simulink model "EMC_no_hand"  (R2015a)
settings: Solver=ode4  SolverMode=MultiTasking  StartTime=0.0  StopTime=inf  FixedStep=BKIN_STEP_TIME  RelTol=1e-3
StartFcn:
  |  warndlg('Dexterit-E models cannot run under simulation. Please compile your model and run it from within Dexterit-E.');set_param(bdroot,'SimulationCommand','stop')
model workspace (MAT data in the model file):
  BKIN_KINEMATIC_FRAME_SIZE = 400
  BKIN_STEP_TIME = 0.00025
  COLOR = 4
  COL_X = 1
  COL_Y = 2
  E_NO_EVENT = 0
  LOAD_X = 1
  LOAD_Y = 2
  MOVEMENT_DELAY = 3
  PATH_LENGTH = 1
  PATH_PERIOD = 2
  POST_TRIAL_DELAY = 4
  RADIUS = 3
  TRAJECTORY = 1
  TRAJECTORY_TYPE = 2
  TRIAL_END = 3
  TRIAL_MOVEMENT = 2
  TRIAL_RESET = 4
  TRIAL_START = 1
  X_POSITION = 1
  Y_POSITION = 2
  col_x = 1
  col_y = 2
  ANGULAR_THRESHOLD = 5
  GAZE_EXIT = 6
  START_REACHED = 7
  FIXATION_DURATION = 6
  TRACKING_TARGET_ROW = 7
  FEEDBACK_COLOR = 5
  CROSS_LOGICAL_RADIUS = 8
  DETECT_FIXATION = 8
  GAZE_IN_TARGET = 5
  START_STABILIZATION = 9
  HAND_IN_TARGET = 9
  BACKGROUND_LOAD = 10
  DIST_BETWEEN_TRAJ = 11
  STRAIGHT_PAUSE_TIME = 12
libraries: simulink x14, xpcrtudplib x12, xpcutilitieslib x10, xpcobsoletelib x8, slrtlib x2, ethercat x2, General x2, Video x2
(part 1 of 6)
settings Model: ModifiedComment=chris -- Wed Feb 16 09:18:30 2005 -- Version 1.1384  ModifiedHistory=Feb 16/05 - Add error repeat, add offset ramp  CovHtmlReporting=off  ExtModeArmWhenConnect=off  ExtModeLogAll=off  Creator=Chris Grebeldinger  LastModifiedBy=Brain and Action Lab
settings SolverCC: EnableConcurrentExecution=on  AutoInsertRateTranBlk=on
settings DataIOCC: LimitDataPoints=off  SignalLoggingSaveFormat=ModelDataLogs  SaveOutput=off  SaveTime=off  SignalLoggingName=sigsOut
settings OptimizationCC: BlockReduction=off  BooleanDataType=off  OptimizeBlockIOStorage=off  BufferReuse=off  GlobalBufferReuse=off  ExpressionFolding=off  ExpressionDepthLimit=2147483647  LocalBlockOutputs=off  InitFltsAndDblsToZero=on
settings DebuggingCC: SaveWithParameterizedLinksMsg=none  UnderspecifiedInitializationDetection=Classic  MergeDetectMultiDrivingBlocksExec=none  SignalResolutionControl=TryResolveAllWithWarning  MultiTaskDSMMsg=warning  FcnCallInpInsideContextMsg=EnableAllAsWarning  StateNameClashWarn=warning  StrictBusMsg=ErrorOnBusTreatedAsVector
settings HardwareCC: ProdIntDivRoundTo=Zero  ProdEndianess=LittleEndian  ProdLongLongMode=on  ProdHWDeviceType=Generic->32-bit x86 compatible  TargetHWDeviceType=32-bit Generic
settings SFSimCC: SimCustomSourceCode=#include <stdlib.h>  SimCustomHeaderCode="#include \"stdlib.h\""  SFSimEcho=off  SimParseCustomCode=off
settings RTWCC: SystemTargetFile=slrt.tlc  TemplateMakefile=slrt_default_tmf  Description=Simulink Real-Time  CustomSourceCode="#include \"stdlib.h\""  CodeExecutionProfiling=on
settings CodeAppCC: MaxIdLength=63
settings SimulinkRealTimeCC: TargetFcnLib=ansi_tfl_tmw.mat  GeneratePreprocessorConditionals=Disable all

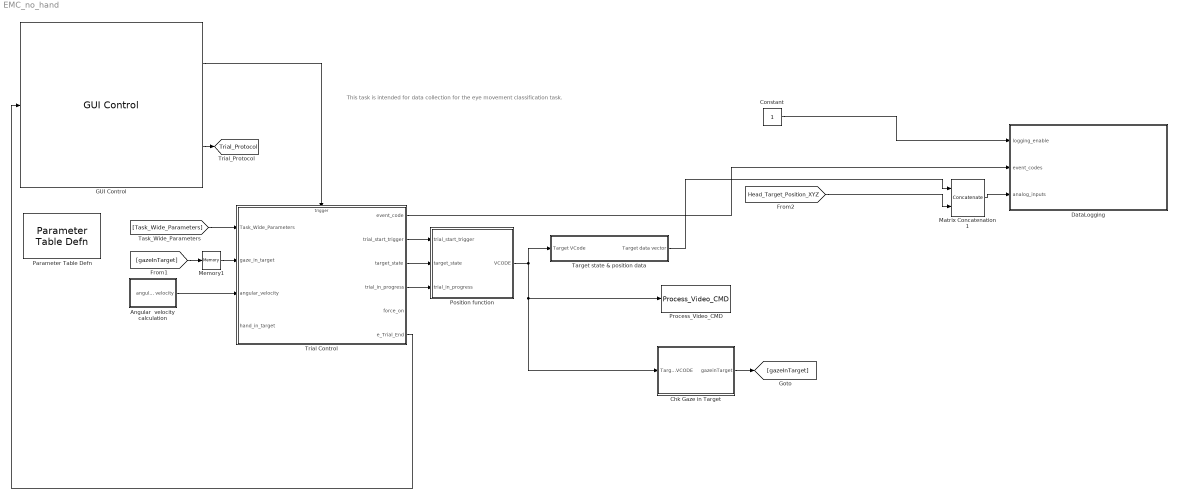
== system EMC_no_hand ==
  note: This task is intended for data collection for the eye movement classification task.
  Angular  velocity calculation : Subsystem
  Chk Gaze in Target : Subsystem
  Constant : Constant
  DataLogging : Subsystem  AncestorBlock=General/DataLogging  mask(DataLogging){log_event_codes=on, log_analog_inputs=on, show_time_remaining=off, ecat_include=on}
      mask prompts: log_event_codes "Log event codes"; log_analog_inputs "Log analog inputs"; show_time_remaining "Show time remaining"; ecat_include "Include EtherCAT control"
      mask help:
      | <b>Do not rename this block, it must be called 'DataLogging'.</b>
      | <p>
      | This block collects the following data and sends it to Dexterit-E:
      | <ul>
      | <li>Robot kinematics</li>
      | <li>Data from KINARM Lab peripherals (optional)</li>
      | <li>Event codes (optional)</li>
      | <li>Programmer supplied data and analog inputs (optional)</li>
      | <li>Remaining task time in seconds (optional)</li>
      | <li>Including code for EtherCAT control system (optional)</li>
      | </lu>
      | <p>
      | This block must be present in all task programs.
      mask init:
      | %this stops us from running a simulation
      | set_param(bdroot,'StartFcn',' warndlg(''Dexterit-E models cannot run under simulation. Please compile your model and run it from within Dexterit-E.'');set_param(bdroot,''SimulationCommand'',''stop'')')
      | 
      | block_path = gcb;  % store block path, as gcb may change with block operations
      |  
      | idxs = findstr(block_path, '/DataLogging');
      | [idxCount, n] = size(idxs);
      | [m, strlen] = size(block_path);
      | bColorSet = 0;
      | 
      | dexcheck();
      | if idxCount == 0 || idxs(1) ~= strlen - 11
      |     fprintf('=========ERROR====================\n');
      |     fprintf('%s should be called DataLogging, attempting to rename.\n', block_path);
      |     try
      |         set_param(block_path, 'Name', 'DataLogging');
      |         block_path = gcb;  % store block path, as gcb may change with block operations
      |         fprintf('Rename successful\n');
      |     catch err
      |         fprintf('Rename failed. You may have 2 DataLogging blocks or another improperly named block.\n');
      |        	set_param(block_path, 'BackgroundColor', '[0.9, 0, 0]');
      |         bColorSet = 1;
      |     end
      |     fprintf('=============================\n');
      | end
      | 
      | log_event_codes = strcmp(get_param(block_path, 'log_event_codes'), 'on');
      | log_analog_inputs = strcmp(get_param(block_path, 'log_analog_inputs'), 'on');
      | show_time_remaining = strcmp(get_param(block_path, 'show_time_remaining'), 'on');
      | 
      | 
      | % Handle the event codes setting: swap the 'Event Codes' inport with a constant block or 
      | % vice versa, if necessary, so that it matches the setting.
      | block_type = get_param([block_path '/event_codes'], 'BlockType');
      |  
      | if log_event_codes && ~strcmp(block_type, 'Inport') || ...  % if a change is required...
      |    ~log_event_codes && strcmp(block_type, 'Inport')
      |     
      |     % ...delete the existing block, ...
      |     pos = get_param([block_path '/event_codes'], 'Position');
      |     delete_line(block_path, 'event_codes/1', 'Create Event Codes Subsystem/1');
      |     delete_block([block_path '/event_codes']);
      |     
      |     % ...add an Inport or a 0-value Constant in place of the previous block (according to
      |     % the new setting), update the signal width flag, and then...
      |     if log_event_codes && ~strcmp(block_type, 'Inport')
      |         add_block('built-in/Inport', [block_path '/event_codes'], 'Name', 'event_codes');
      |         set_param([block_path '/Create Event Codes Subsystem/Not Logging Event Codes'], 'Value', '0');
      |     else
      |         add_block('built-in/Constant', [block_path '/event_codes'], 'Name', 'event_codes');
      |         set_param([block_path '/event_codes'], 'Value', '0');
      |         set_param([block_path '/Create Event Codes Subsystem/Not Logging Event Codes'], 'Value', '1');
      |     end
      |     
      |     % ...connect the new block.
      |     set_param([block_path '/event_codes'], 'Position', pos);
      |     add_line(block_path, 'event_codes/1', 'Create Event Codes Subsystem/1');
      | end
      | 
      | % Swap the 'analog_data' inport with a constant block or vice versa according to the corresponding setting.
      | block_type = get_param([block_path '/analog_inputs'], 'BlockType');
      | 
      | if log_analog_inputs && ~strcmp(block_type, 'Inport') || ...  % if a change is required...
      |    ~log_analog_inputs && strcmp(block_type, 'Inport')
      |     
      |     % ...delete the existing block, ...
      |     pos = get_param([block_path '/analog_inputs'], 'Position');
      |     delete_line(block_path, 'analog_inputs/1', 'Create Analog Inputs Subsystem/1');
      |     delete_block([block_path '/analog_inputs']);
      |     
      |     % ...add an Inport or a 0-value Constant in place of the previous block (according to
      |     % the new setting), update the signal width flag, and then...
      |     if log_analog_inputs && ~strcmp(block_type, 'Inport')
      |         add_block('built-in/Inport', [block_path '/analog_inputs'], 'Name', 'analog_inputs');
      |         set_param([block_path '/Create Analog Inputs Subsystem/Not Logging Analog Inputs'], 'Value', '0');
      |     else
      |         add_block('built-in/Constant', [block_path '/analog_inputs'], 'Name', 'analog_inputs');
      |         set_param([block_path '/analog_inputs'], 'Value', '0');
      |         set_param([block_path '/Create Analog Inputs Subsystem/Not Logging Analog Inputs'], 'Value', '1');
      |     end
      |     
      |     % ...connect the new block.
      |     set_param([block_path '/analog_inputs'], 'Position', pos);
      |     add_line(block_path, 'analog_inputs/1', 'Create Analog Inputs Subsystem/1');
      | end
      | 
      | %%%%%%%%%%%%%%%%%%%%%%%%%%%%%%%%%%%%%%%%%%%%%
      | block_type = get_param([block_path '/seconds_remaining'], 'BlockType');
      |  
      | if show_time_remaining && ~strcmp(block_type, 'Inport') || ...  % if a change is required...
      |    ~show_time_remaining && strcmp(block_type, 'Inport')
      |     
      |     % ...delete the existing block, ...
      |     pos = get_param([block_path '/seconds_remaining'], 'Position');
      |     delete_line(block_path, 'seconds_remaining/1', 'Create Custom Data Subsystem/1');
      |     delete_block([block_path '/seconds_remaining']);
      |     
      |     % ...add an Inport or a 0-value Constant in place of the previous block (according to
      |     % the new setting), update the signal width flag, and then...
      |     if show_time_remaining && ~strcmp(block_type, 'Inport')
      |         add_block('built-in/Inport', [block_path '/seconds_remaining'], 'Name', 'seconds_remaining');
      |     else
      |         add_block('built-in/Constant', [block_path '/seconds_remaining'], 'Name', 'seconds_remaining');
      |         set_param([block_path '/seconds_remaining'], 'Value', '-1');
      |     end
      |     
      |     % ...connect the new block.
      |     set_param([block_path '/seconds_remaining'], 'Position', pos);
      |     add_line(block_path, 'seconds_remaining/1', 'Create Custom Data Subsystem/1');
      | end
      | %%%%%%%%%%%%%%%%%%%%%%%%%%%%%%%%%%%%%%%%%%%%%%%%%%%%%%%%%
      | 
      | % Create the text label for the block, and use it to create the first in a 
      | % list of drawing commands that will be used to draw the mask icon.
      | label = 'Logging:\n ';
      |  
      | if log_event_codes
      |    label = [label 'Event codes\n'];
      | end
      |  
      | label = [label 'KINARM data\n'];
      |     
      | if log_analog_inputs
      |     label = [label 'Analog inputs\n'];
      | end
      | 
      | if show_time_remaining
      |     label = [label 'Seconds remaining\n'];
      | end
      | 
      | draw_commands = 'disp(label); ';
      | 
      | % Ensure the inports appear in a fixed order, and for each inport found add
      | % to the list of drawing commands a command to label it.
      | inports = find_system(block_path, 'LookUnderMasks', 'all', 'FollowLinks', 'on', 'SearchDepth', 1, 'BlockType', 'Inport');
      | 
      | for i = 1:length(inports)
      |     inport_name = char(get_param(inports(i), 'Name'));
      |     
      |     if strcmp(inport_name, 'logging_enable')
      |         port = '1';
      |     elseif strcmp(inport_name, 'event_codes')
      |         port = '2';
      |     elseif strcmp(inport_name, 'analog_inputs')
      |         if log_event_codes
      |             port = '3';
      |         else
      |             port = '2';
      |         end
      |     elseif strcmp(inport_name, 'seconds_remaining')
      |         if log_event_codes && log_analog_inputs
      |             port = '4';
      |         elseif log_event_codes || log_analog_inputs
      |             port = '3';
      |         else
      |             port = '2';                
      |         end
      |     end
      |     
      |     set_param([block_path '/' inport_name], 'Port', port);
      |     draw_commands = [draw_commands 'port_label(''input'', ' port ', ''' inport_name '''); '];
      | end
      | 
      | % Apply the drawing commands.
      | set_param(block_path, 'MaskDisplay', draw_commands);
      | 
      | %%% Handle background colours if link status changes.  
      | checkBackgroundColour(block_path, 'General');
      | 
      | % For gaze tracking, the packet length is variable, so we need to check off that option the Receive UDP block.
      | %set_param([block_path '/Receive_Gaze/Receive'], 'vblLen', 'on')
      | 
      | updateUDP([block_path '/Network Transfer Subsystem/UDP Receiver']);
      | initPollKINARM(ecat_include);
      settings: PostSaveFcn=|
      | name_size = strfind(gcb, '/') - 1;
      | if name_size > 50
      |   warndlg('The given file name is longer than 50 characters. The task name will be truncated in Dexterit-E.')
      | end
      mask Help:
      | Sends task progress, kinematics, analog data and event codes to Dexterit-E.
      | 
      | <H2>Library </H2>
      | General
      | 
      | <H2>Description </H2>
      | <b>Do not rename this block, it must be called 'DataLogging'.</b>
      | <p>
      | The DataLogging block collects data and event codes and sends it to Dexterit-E for saving.  It also passes on Task Program information that is invisible to the user, and so must be present even if no data is going to be saved.
      | <P>
      | <B><I>This block must be present in all Task Programs, even if no data is going to be saved.</I></B>
      | 
      | 
      | <H2>Parameters and Dialog Box</H2>
      | <ul><li><B>Log event codes: </B> checking this parameter causes the Dexterit-E to log event codes specified by the event_codes input.
      | Event codes are only saved at 1 kHz. If you need to save event codes at a higher rate then you will need to send an array of values to the event_codes input.
      | </li>
      | <li><B>Log analog inputs: </B> checking this parameter causes Dexterit-E to log analog data specified by the analog_inputs input.
      | Analog data in this context can be any numbers you would like to save. The data can truly be analog data from a card like the NI-6229,
      | but it can also be calculations created during your model's execution. For example, if you move targets around the screen then it
      | can be useful to send the target X, Y positions out as 2 separate "analog channels".
      | </li>
      | <li><B>Show time remaining: </B> checking this parameter causes Dexterit-E to display the number of seconds remaining in the task as specified by the seconds_remaining input
      | </li>
      | <li><b>Include EtherCAT control: </b>KINARM labs have one of two different control systems: PMAC or EtherCAT. If your KINARM uses the PMAC control system AND you are not planning to run your task on KINARMs that use the EtherCAT control system then you can uncheck this box. You can find out which control system your KINARM uses by looking in Dexterit-E at the "KINARM Lab components" dialog. Unchecking this box should reduce your compile times. This box only affects MATLAB version 2015a SP1 and later.
      | </li>
      | </ul>
      | <p>
      | <ul><li><B>analog_inputs: </B> this vector input specifies the data from analog inputs and other arbitrary data to be logged by Dexterit-E.
      | </li>
      | <li><B>event_codes: </B> this input should be a vector of 16 bit integers.  These event codes are passed to Dexterit-E, which saves the integers as event codes (i.e. they are timestamped so that events that occurred duing a task can be related to the other saved data).
      | </li>
      | <li><B>logging_enable: </B> this input is used by Dexterit-E to indicate when to save data.  When logging_enable is 1, data is saved.  When logging_enable is 0, data is not saved.  (Note: data saving is also affected by the Run/Pause button in Dexterit-E.  When the task is paused, data is no longer saved regardless of the value of this input).
      | </li>
      | <li><B>seconds_remaining: </B> this input is used by Dexterit-E to update the number of seconds remaining in the task. If this is not supplied then 'n/a' is displayed.
      | </li>
      | </ul>
      mask Display: disp(label); port_label('input', 1, 'logging_enable'); port_label('input', 2, 'event_codes'); port_label('input', 3, 'analog_inputs');
  GUI Control : General/GUI Control  task_version=1.0  show_repeat_trial_flag=off  use_custom_tp=off  target_type_str=Circle  Target_Type=1  XYcols=[1 2]  Vcols=3  Lcols=4  indices_padding=[0 0 0 0;0 0 0 0]  target_table_rows=64  load_table_rows=20  tp_table_rows=100
  Matrix Concatenation1 : Concatenate
  Memory1 : Memory
  Parameter Table Defn : General/Parameter Table Defn  ShowInLibBrowser=0
  Position function : Subsystem
  Process_Video_CMD : Video/Process_Video_CMD  video_delay=50
  Target state & position data : Subsystem
  Trial Control : Stateflow chart  TreatAsAtomicUnit=on
  tag scope: Trial_Protocol=global
  wires:
  GUI Control/1 -> Trial Control/Trigger
  Position function/1(VCODE) -> Chk Gaze in Target/1(Target VCODE), Process_Video_CMD/1, Target state & position data/1(Target VCode)
  Trial Control/6(e_Trial_End) -> GUI Control/1
  Trial Control/2(trial_start_trigger) -> Position function/1(trial_start_trigger)
  [Task_Wide_Parameters] -> Trial Control/1(Task_Wide_Parameters)
  GUI Control/2 -> [Trial_Protocol]
  Trial Control/3(target_state) -> Position function/2(target_state)
  Trial Control/4(trial_in_progress) -> Position function/3(trial_in_progress)
  Trial Control/1(event_code) -> DataLogging/2(event_codes)
  Target state & position data/1(Target data vector) -> Matrix Concatenation1/1
  Angular  velocity calculation/1(angular velocity) -> Trial Control/3(angular_velocity)
  [gazeInTarget] -> Memory1/1
  Memory1/1 -> Trial Control/2(gaze_in_target)
  Chk Gaze in Target/1(gazeinTarget) -> [gazeInTarget]
  Constant/1 -> DataLogging/1(logging_enable)
  Matrix Concatenation1/1 -> DataLogging/3(analog_inputs)
  [Head_Target_Position_XYZ] -> Matrix Concatenation1/2

== system EMC_no_hand/Angular  velocity calculation ==
  Gaze angular velocity : MATLAB Function  TreatAsAtomicUnit=on
  Memory4 : Memory
  angular velocity : Outport
  wires:
  Gaze angular velocity/1(angularVelocity) -> angular velocity/1
  Memory4/1 -> Gaze angular velocity/1(gazeData)
  [Gaze_Global] -> Memory4/1

== system EMC_no_hand/Chk Gaze in Target ==
  Target VCODE : Inport
  Cross Vector : Selector  Indices=[1 2 3 4 10]
  Data Type Conversion : DataTypeConversion  OutDataTypeStr=boolean
  Gaze Selector : Selector  Indices=[1 2]
  MATLAB Function : MATLAB Function  TreatAsAtomicUnit=on
  "Scope (xPC) " : slrtlib/Displays and Logging/Scope   scopeno=2  scopetype=Target  autostart=on  viewmode=Numerical  formatstr='%15.6f'  grid=on  ylimits=[0,0]  nosamples=250  noprepostsamples=0  interleave=1  triggermode=FreeRun  triggersignal=1  trigsignalfromport=off  triggerlevel=0.0  triggerslope=Either  triggerscope=1  triggersample=0  filename=data.dat  mode=Lazy  writesize=512  autorestart=off  dynamicfilemode=off  maxwritefilesize=512*1024^2
  Scope (xPC) 2 : slrtlib/Displays and Logging/Scope   scopeno=1  scopetype=Target  autostart=on  viewmode=Numerical  formatstr='%15.6f'  grid=on  ylimits=[0,0]  nosamples=250  noprepostsamples=0  interleave=1  triggermode=FreeRun  triggersignal=1  trigsignalfromport=off  triggerlevel=0.0  triggerslope=Either  triggerscope=1  triggersample=0  filename=data.dat  mode=Lazy  writesize=512  autorestart=off  dynamicfilemode=off  maxwritefilesize=512*1024^2
  Selector : Selector  Indices=CROSS_LOGICAL_RADIUS
  gazeinTarget : Outport
  wires:
  Gaze Selector/1 -> "Scope (xPC) "/1, MATLAB Function/1(gaze)
  [Gaze_Global] -> Gaze Selector/1
  Target VCODE/1 -> Cross Vector/1
  MATLAB Function/1(gaze_in_target) -> Data Type Conversion/1
  Cross Vector/1 -> MATLAB Function/2(target)
  Data Type Conversion/1 -> gazeinTarget/1
  MATLAB Function/2(dist) -> Scope (xPC) 2/1
  [Task_Wide_Parameters] -> Selector/1
  Selector/1 -> MATLAB Function/3(logical_radius)

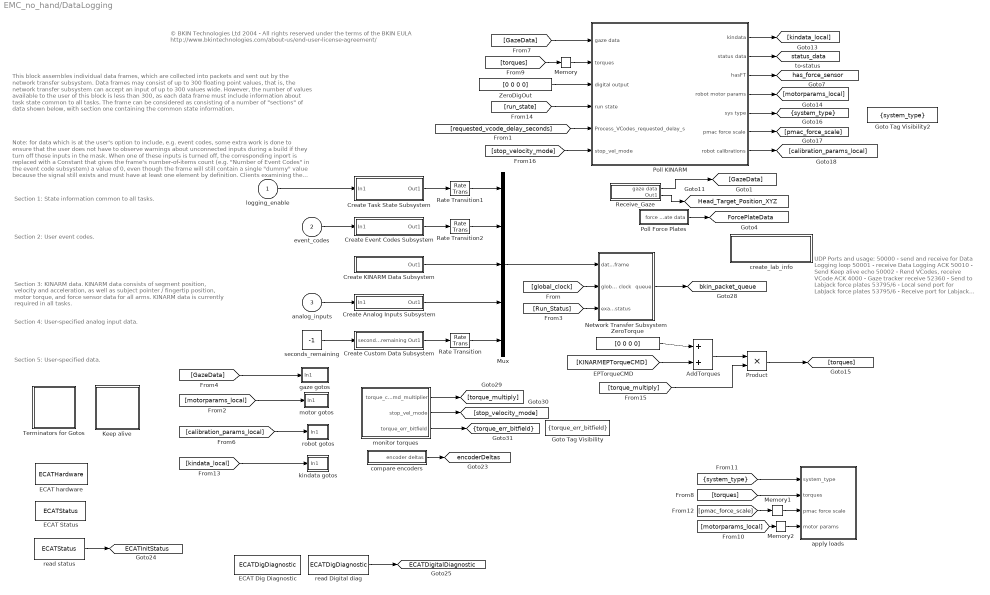
== system EMC_no_hand/DataLogging ==
  note: UDP Ports and usage:
      | 50000 - send and receive for Data Logging loop
      | 50001 - receive Data Logging ACK
      | 50010 - Send Keep alive echo
      | 50002 - Rend VCodes, receive VCode ACK
      |
      | 4000 - Gaze tracker receive
      | 52360 - Send to Labjack force plates
      | 53795/6 - Local send port for LabJack force plates
      | 53795/6 - Receive port for Labjack Force plates
  note: Section 5: User-specified data.
  note: Note: for data which is at the user's option to include, e.g. event codes, some extra work is done to ensure that the user
      | does not have to observe warnings about unconnected inputs during a build if they turn off those inputs in the mask. When
      | one of these inputs is turned off, the corresponding inport is replaced with a Constant that gives the frame's number-of-items
      | count (e.g. "Number of Event Codes" in the event code subsystem) a value of 0, even though the frame will still contain a
      | single "dummy" value because the signal still exists and must have at least one element by definition. Clients examining the
      | data frames must be aware of this and ignore the dummy value.
      |
      | If a user opts to keep the inport available but connects nothing to it, Simulink resolves that as a single signal with value 0.
  note: Section 3: KINARM data. KINARM data consists of segment
      | position, velocity and acceleration, as well as subject pointer /
      | fingertip position, motor torque, and force sensor data for all arms.
      | KINARM data is currently required in all tasks.
  note: Section 2: User event codes.
  note: Section 1: State information common to all tasks.
  note: Section 4: User-specified analog input data.
  note: This block assembles individual data frames, which are collected into packets and sent out by the network transfer subsystem.
      |
      | Data frames may consist of up to 300 floating point values, that is, the network transfer subsystem can accept an input of up
      | to 300 values wide. However, the number of values available to the user of this block is less than 300, as each data frame
      | must include information about task state common to all tasks. The frame can be considered as consisting of a number of
      | "sections" of data shown below, with section one containing the common state information.
  note: © BKIN Technologies Ltd 2004  - All rights reserved under the terms of the BKIN EULA
      | http://www.bkintechnologies.com/about-us/end-user-license-agreement/
  logging_enable : Inport
  event_codes : Inport  Port=2
  analog_inputs : Inport  Port=3
  AddTorques : Sum
  Create Analog Inputs Subsystem : Subsystem
  Create Custom Data Subsystem : Subsystem
  Create Event Codes Subsystem : Subsystem
  Create KINARM Data Subsystem : Subsystem
  Create Task State Subsystem : Subsystem
  ECAT Dig Diagnostic : DataStoreMemory  DataStoreName=ECATDigDiagnostic  ReadBeforeWriteMsg=error  WriteAfterWriteMsg=warning  WriteAfterReadMsg=error  InitialValue=zeros(1,4)  OutDataTypeStr=uint32
  ECAT Status : DataStoreMemory  DataStoreName=ECATStatus  ReadBeforeWriteMsg=error  WriteAfterWriteMsg=warning  WriteAfterReadMsg=error  InitialValue=zeros(1,8)  OutDataTypeStr=double
  ECAT hardware : DataStoreMemory  DataStoreName=ECATHardware  ReadBeforeWriteMsg=error  WriteAfterWriteMsg=warning  WriteAfterReadMsg=error  InitialValue=zeros(1,14)  OutDataTypeStr=double
  Goto Tag Visibility : GotoTagVisibility  GotoTag=torque_err_bitfield
  Goto Tag Visibility2 : GotoTagVisibility  GotoTag=system_type
  Keep alive : Subsystem  TreatAsAtomicUnit=on
      settings: RTWSystemCode=Nonreusable function  RTWFileNameOpts=Use function name
  Memory : Memory
  Memory1 : Memory
  Memory2 : Memory
  Mux : Mux  Inputs=5
  Network Transfer Subsystem : Subsystem  TreatAsAtomicUnit=on
      settings: RTWSystemCode=Nonreusable function  RTWFileNameOpts=Use function name
  Poll Force Plates : Subsystem  TreatAsAtomicUnit=on
      settings: RTWSystemCode=Nonreusable function  RTWFileNameOpts=Use function name
  Poll KINARM : Subsystem  TreatAsAtomicUnit=on
      settings: RTWSystemCode=Nonreusable function  RTWFileNameOpts=Use function name
  Product : Product
  Rate Transition : RateTransition  Integrity=off
  Rate Transition1 : RateTransition  Integrity=off
  Rate Transition2 : RateTransition  Integrity=off
  Receive_Gaze : Subsystem  TreatAsAtomicUnit=on
      settings: RTWSystemCode=Nonreusable function  RTWFileNameOpts=Use function name
  Terminators for Gotos : Subsystem
  ZeroDigOut : Constant  Value=[0 0 0 0]
  ZeroTorque : Constant  Value=[0 0 0 0]
  apply loads : Subsystem  TreatAsAtomicUnit=on
      settings: RTWSystemCode=Nonreusable function  RTWFileNameOpts=Use function name
  compare encoders : Subsystem
  create_lab_info : Subsystem
  gaze gotos : Subsystem
  kindata gotos : Subsystem
  monitor torques : Subsystem
  motor gotos : Subsystem
  read Digital diag : DataStoreRead  DataStoreName=ECATDigDiagnostic  SampleTime=BKIN_STEP_TIME
  read status : DataStoreRead  DataStoreName=ECATStatus  SampleTime=BKIN_STEP_TIME
  robot gotos : Subsystem
  seconds_remaining : Constant  Value=-1
  tag scope: ECATDigitalDiagnostic=global, ECATInitStatus=global, ForcePlateData=global, Head_Target_Position_XYZ=global, bkin_packet_queue=global, encoderDeltas=global, has_force_sensor=global, status_data=global, system_type=scoped, torque_err_bitfield=scoped
  wires:
  [stop_velocity_mode] -> Poll KINARM/6(stop_vel_mode)
  monitor torques/3(torque_err_bitfield) -> [torque_err_bitfield]
  monitor torques/2(stop_vel_mode) -> [stop_velocity_mode]
  monitor torques/1(torque_cmd_multiplier) -> [torque_multiply]
  Product/1 -> [torques]
  [torque_multiply] -> Product/2
  AddTorques/1 -> Product/1
  [kindata_local] -> kindata gotos/1(In1)
  [calibration_params_local] -> robot gotos/1(In1)
  [motorparams_local] -> motor gotos/1(In1)
  [GazeData] -> gaze gotos/1(In1)
  seconds_remaining/1 -> Create Custom Data Subsystem/1(second_remaining)
  Poll KINARM/3(hasFT) -> [has_force_sensor]
  Poll KINARM/2(status data) -> [status_data]
  [Run_Status] -> Network Transfer Subsystem/3(exam_status)
  [global_clock] -> Network Transfer Subsystem/2(global clock)
  Poll Force Plates/1(force plate data) -> [ForcePlateData]
  Rate Transition2/1 -> Mux/2
  Create Custom Data Subsystem/1(Out1) -> Rate Transition/1
  Create Analog Inputs Subsystem/1(Out1) -> Mux/4
  Create KINARM Data Subsystem/1(Out1) -> Mux/3
  Create Event Codes Subsystem/1(Out1) -> Rate Transition2/1
  Create Task State Subsystem/1(Out1) -> Rate Transition1/1
  logging_enable/1 -> Create Task State Subsystem/1(In1)
  Mux/1 -> Network Transfer Subsystem/1(data_frame)
  Rate Transition/1 -> Mux/5
  Rate Transition1/1 -> Mux/1
  Poll KINARM/1(kindata) -> [kindata_local]
  Poll KINARM/4(robot motor params) -> [motorparams_local]
  [GazeData] -> Poll KINARM/1(gaze data)
  [torques] -> apply loads/2(torques)
  [torques] -> Memory/1
  Memory/1 -> Poll KINARM/2(torques)
  [motorparams_local] -> Memory2/1
  Poll KINARM/5(sys type) -> [system_type]
  [system_type] -> apply loads/1(system_type)
  Poll KINARM/6(pmac force scale) -> [pmac_force_scale]
  [pmac_force_scale] -> Memory1/1
  Memory1/1 -> apply loads/3(pmac force scale)
  Memory2/1 -> apply loads/4(motor params)
  Poll KINARM/7(robot calibrations) -> [calibration_params_local]
  ZeroDigOut/1 -> Poll KINARM/3(digital output)
  compare encoders/1(encoder deltas) -> [encoderDeltas]
  [run_state] -> Poll KINARM/4(run state)
  read status/1 -> [ECATInitStatus]
  read Digital diag/1 -> [ECATDigitalDiagnostic]
  [requested_vcode_delay_seconds] -> Poll KINARM/5(Process_VCodes_requested_delay_s)
  Network Transfer Subsystem/1(queue) -> [bkin_packet_queue]
  ZeroTorque/1 -> AddTorques/1
  event_codes/1 -> Create Event Codes Subsystem/1(In1)
  analog_inputs/1 -> Create Analog Inputs Subsystem/1(In1)
  [KINARMEPTorqueCMD] -> AddTorques/2
  Receive_Gaze/1(gaze data) -> [GazeData]
  Receive_Gaze/2(Out1) -> [Head_Target_Position_XYZ]

== system EMC_no_hand/Position function ==
  trial_start_trigger : Inport
  target_state : Inport  Port=2
  trial_in_progress : Inport  Port=3
  Constant : Constant
  MATLAB Function : MATLAB Function  TreatAsAtomicUnit=on
  Main/Start target VCODE2 : MATLAB Function  TreatAsAtomicUnit=on
  Selector : Selector  Indices=PATH_PERIOD
  Selector1 : Selector  Indices=PATH_LENGTH
  Selector2 : Selector  Indices=TRAJECTORY
  Selector3 : Selector  Indices=TRAJECTORY_TYPE
  Selector4 : Selector  Indices=DIST_BETWEEN_TRAJ
  Selector5 : Selector  Indices=STRAIGHT_PAUSE_TIME
  Show_Target : Video/Show_Target  target_type=Circle  num_states=2  attribcol1=[4 4 0 3]  attribcol2=[5 5 0 3]  attribcol3=[0 0 0 0]  attribcol4=[0 0 0 0]  attribcol5=[0 0 0 0]  stateindices_padding=[0 0 0 0 0 0 0;0 0 0 0 0 0 0;0 0 0 0 0 0 0;0 0 0 0 0 0 0;0 0 0 0 0 0 0]  source=dialog  opacity=100  target_display=Both subject and operator displays  num_col=4
  VCODE : Outport  PortDimensions=[1,70]
  wires:
  Main/Start target VCODE2/1(outTargetVCode) -> VCODE/1
  trial_start_trigger/1 -> Main/Start target VCODE2/9(trialStartTrigger)
  [Task_Wide_Parameters] -> Selector4/1, Selector5/1, Selector1/1, Selector/1
  Selector/1 -> Main/Start target VCODE2/6(pathPeriod)
  Selector1/1 -> Main/Start target VCODE2/5(pathLength)
  Show_Target/1 -> Main/Start target VCODE2/10(inTargetVCode)
  Constant/1 -> Show_Target/1
  Selector2/1 -> Main/Start target VCODE2/11(inTrajectory)
  [Trial_Protocol] -> Selector3/1, Selector2/1
  target_state/1 -> Show_Target/2
  trial_in_progress/1 -> Main/Start target VCODE2/1(trialInProgress)
  Selector3/1 -> Main/Start target VCODE2/12(inTrajectoryType)
  MATLAB Function/1(pseudorandom_trajectory_parameters) -> Main/Start target VCODE2/2(pseudorandom_table)
  MATLAB Function/2(diagonal_trajectory_parameters) -> Main/Start target VCODE2/3(diagonal_table)
  MATLAB Function/3(sinusoidal_trajectory_parameters) -> Main/Start target VCODE2/4(sinusoidal_table)
  Selector4/1 -> Main/Start target VCODE2/8(distanceBetweenTrajectories)
  Selector5/1 -> Main/Start target VCODE2/7(straightPauseTime)

== system EMC_no_hand/Target state & position data ==
  Target VCode : Inport
  MATLAB Function1 : MATLAB Function  TreatAsAtomicUnit=on
  Mux : Mux  Inputs=3
  Target data vector : Outport
  wires:
  Mux/1 -> Target data vector/1
  Target VCode/1 -> MATLAB Function1/1(targetVCode)
  MATLAB Function1/2(targetX) -> Mux/2
  MATLAB Function1/1(targetOn) -> Mux/1
  MATLAB Function1/3(targetY) -> Mux/3

== system EMC_no_hand/DataLogging/Create Analog Inputs Subsystem ==
  In1 : Inport
  Analog Data Width : DataTypeConversion  SaturateOnIntegerOverflow=on  RndMeth=Zero
  Mux2 : Mux  Inputs=2
  Not Logging Analog Inputs : Constant  Value=0
  Rate Transition : RateTransition  Integrity=off
  Subtract : Sum  Inputs=-+
  Width : Width
  Out1 : Outport
  wires:
  Rate Transition/1 -> Out1/1
  Mux2/1 -> Analog Data Width/1
  Analog Data Width/1 -> Rate Transition/1
  Not Logging Analog Inputs/1 -> Subtract/1
  Width/1 -> Subtract/2
  Subtract/1 -> Mux2/1
  In1/1 -> Width/1, Mux2/2

== system EMC_no_hand/DataLogging/Create Custom Data Subsystem ==
  second_remaining : Inport
  Mux1 : Mux  Inputs=6
  Mux6 : Mux  Inputs=2
  Rate Transition1 : RateTransition  Integrity=off
  Rate Transition2 : RateTransition  Integrity=off
  Width : Width
  custom_version : Constant  Value=8  OutDataTypeStr=double
  Out1 : Outport
  wires:
  [torque_err_bitfield] -> Mux1/6
  Mux6/1 -> Out1/1
  Mux1/1 -> Mux6/2, Width/1
  Width/1 -> Mux6/1
  custom_version/1 -> Mux1/1
  [status_data] -> Mux1/2
  [encoderDeltas] -> Mux1/3
  Rate Transition1/1 -> Mux1/4
  second_remaining/1 -> Rate Transition1/1
  [vcode_error] -> Rate Transition2/1
  Rate Transition2/1 -> Mux1/5

== system EMC_no_hand/DataLogging/Create Event Codes Subsystem ==
  In1 : Inport
  Event Codes : DataTypeConversion  SaturateOnIntegerOverflow=on  RndMeth=Zero
  Mux4 : Mux  Inputs=2
  Not Logging Event Codes : Constant  Value=0
  Number of Event Codes : DataTypeConversion  SaturateOnIntegerOverflow=on  RndMeth=Zero
  Subtract : Sum  Inputs=-+
  Width : Width
  Out1 : Outport
  wires:
  Mux4/1 -> Out1/1
  In1/1 -> Event Codes/1, Width/1
  Not Logging Event Codes/1 -> Subtract/1
  Subtract/1 -> Number of Event Codes/1
  Width/1 -> Subtract/2
  Number of Event Codes/1 -> Mux4/1
  Event Codes/1 -> Mux4/2

== system EMC_no_hand/DataLogging/Create KINARM Data Subsystem ==
  Bus Selector1 : BusSelector  OutputSignals=Robot1.a1_motor_status,Robot2.a2_motor_status,Robot1.a1_ecatCurrentLimitEnabled,Robot2.a2_ecatCurrentLimitEnabled,Robot1.a1_ep_grip_sensor,Robot2.a2_ep_grip_sensor  OutputAsBus=on
  Bus to Vector1 : BusToVector
  Mux1 : Mux  Inputs=2
  Mux3 : Mux
  Rate Transition : RateTransition  Integrity=off
  Width : Width
  bitfield : MATLAB Function  TreatAsAtomicUnit=on
  gaze_data : Subsystem
  select KINData : Subsystem
  touint : DataTypeConversion  OutDataTypeStr=uint32  SaturateOnIntegerOverflow=on  RndMeth=Zero
  touint1 : DataTypeConversion  OutDataTypeStr=double  SaturateOnIntegerOverflow=on  RndMeth=Zero
  Out1 : Outport
  wires:
  Rate Transition/1 -> Width/1, Mux1/2
  Mux1/1 -> Out1/1
  select KINData/1(Out1) -> Mux3/1
  Width/1 -> Mux1/1
  Mux3/1 -> Rate Transition/1
  gaze_data/1(gaze_channels) -> Mux3/2
  [ForcePlateData] -> Mux3/3
  [KINdata_bus] -> Bus Selector1/1
  Bus Selector1/1 -> Bus to Vector1/1
  Bus to Vector1/1 -> touint/1
  bitfield/1(bitfield) -> touint1/1
  touint/1 -> bitfield/1(motorStatus)
  touint1/1 -> Mux3/4

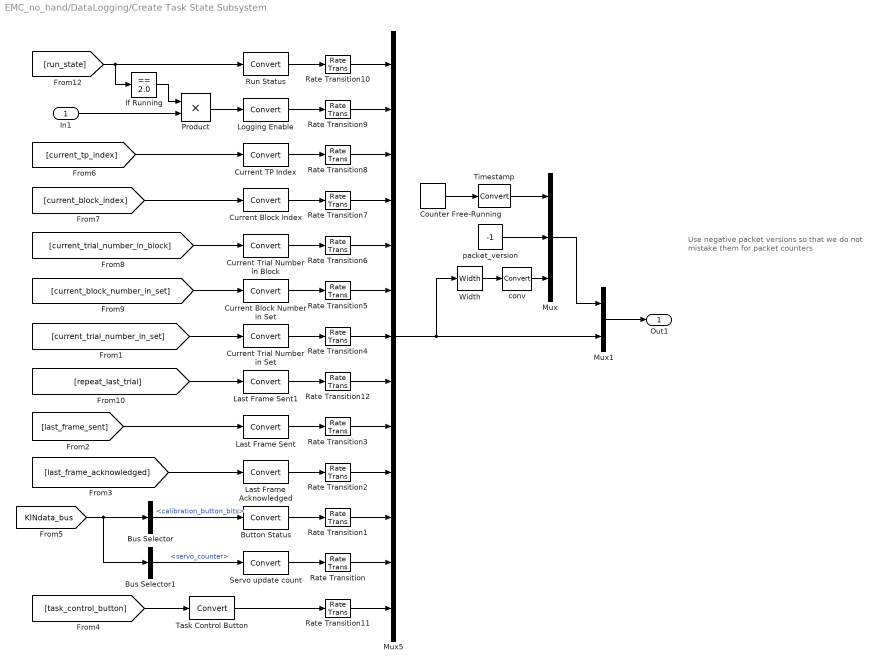
== system EMC_no_hand/DataLogging/Create Task State Subsystem ==
  note: Use negative packet versions so that we do not
      | mistake them for packet counters
  In1 : Inport
  Bus Selector : BusSelector  OutputSignals=KINDataGeneral.calibration_button_bits
  Bus Selector1 : BusSelector  OutputSignals=KINDataGeneral.servo_counter
  Button Status : DataTypeConversion  SaturateOnIntegerOverflow=on  RndMeth=Zero
  Counter Free-Running : simulink/Sources/Counter Free-Running  NumBits=32  tsamp=-1
  Current Block Index : DataTypeConversion  SaturateOnIntegerOverflow=on  RndMeth=Zero
  Current Block Number in Set : DataTypeConversion  SaturateOnIntegerOverflow=on  RndMeth=Zero
  Current TP Index : DataTypeConversion  SaturateOnIntegerOverflow=on  RndMeth=Zero
  Current Trial Number in Block : DataTypeConversion  SaturateOnIntegerOverflow=on  RndMeth=Zero
  Current Trial Number in Set : DataTypeConversion  SaturateOnIntegerOverflow=on  RndMeth=Zero
  If Running : simulink/Logic and Bit Operations/Compare To Constant  relop===  const=2.0  OutDataTypeStr=uint8  ZeroCross=off
  Last Frame Acknowledged : DataTypeConversion  SaturateOnIntegerOverflow=on  RndMeth=Zero
  Last Frame Sent : DataTypeConversion  SaturateOnIntegerOverflow=on  RndMeth=Zero
  Last Frame Sent1 : DataTypeConversion  SaturateOnIntegerOverflow=on  RndMeth=Zero
  Logging Enable : DataTypeConversion  SaturateOnIntegerOverflow=on  RndMeth=Zero
  Mux : Mux  Inputs=3
  Mux1 : Mux  Inputs=2
  Mux5 : Mux  Inputs=13
  Product : Product  RndMeth=Zero
  Rate Transition{,1..12} (13 alike) : RateTransition
  Run Status : DataTypeConversion  SaturateOnIntegerOverflow=on  RndMeth=Zero
  Servo update count : DataTypeConversion  SaturateOnIntegerOverflow=on  RndMeth=Zero
  Task Control Button : DataTypeConversion  SaturateOnIntegerOverflow=on  RndMeth=Zero
  Timestamp : DataTypeConversion  SaturateOnIntegerOverflow=on  RndMeth=Zero
  Width : Width
  conv : DataTypeConversion  SaturateOnIntegerOverflow=on  RndMeth=Zero
  packet_version : Constant  Value=-1
  Out1 : Outport
  wires:
  Rate Transition/1 -> Mux5/12
  Rate Transition1/1 -> Mux5/11
  Rate Transition2/1 -> Mux5/10
  Rate Transition3/1 -> Mux5/9
  Rate Transition12/1 -> Mux5/8
  Rate Transition4/1 -> Mux5/7
  Rate Transition5/1 -> Mux5/6
  Rate Transition6/1 -> Mux5/5
  Rate Transition7/1 -> Mux5/4
  Rate Transition8/1 -> Mux5/3
  Rate Transition9/1 -> Mux5/2
  Rate Transition10/1 -> Mux5/1
  packet_version/1 -> Mux/2
  Timestamp/1 -> Mux/1
  conv/1 -> Mux/3
  Mux1/1 -> Out1/1
  Mux/1 -> Mux1/1
  Mux5/1 -> Mux1/2, Width/1
  Width/1 -> conv/1
  [repeat_last_trial] -> Last Frame Sent1/1
  Last Frame Sent1/1 -> Rate Transition12/1
  Rate Transition11/1 -> Mux5/13
  Task Control Button/1 -> Rate Transition11/1
  [task_control_button] -> Task Control Button/1
  Button Status/1 -> Rate Transition1/1
  [last_frame_acknowledged] -> Last Frame Acknowledged/1
  [last_frame_sent] -> Last Frame Sent/1
  Last Frame Acknowledged/1 -> Rate Transition2/1
  Last Frame Sent/1 -> Rate Transition3/1
  In1/1 -> Product/2
  Current Trial Number in Set/1 -> Rate Transition4/1
  Current Block Number in Set/1 -> Rate Transition5/1
  Current Trial Number in Block/1 -> Rate Transition6/1
  Current Block Index/1 -> Rate Transition7/1
  Current TP Index/1 -> Rate Transition8/1
  Logging Enable/1 -> Rate Transition9/1
  Run Status/1 -> Rate Transition10/1
  [current_trial_number_in_set] -> Current Trial Number in Set/1
  [current_block_number_in_set] -> Current Block Number in Set/1
  [current_trial_number_in_block] -> Current Trial Number in Block/1
  [current_block_index] -> Current Block Index/1
  [current_tp_index] -> Current TP Index/1
  If Running/1 -> Product/1
  Counter Free-Running/1 -> Timestamp/1
  [run_state] -> If Running/1, Run Status/1
  Product/1 -> Logging Enable/1
  Servo update count/1 -> Rate Transition/1
  Bus Selector1/1 -> Servo update count/1  "<servo_counter>"
  [KINdata_bus] -> Bus Selector/1, Bus Selector1/1
  Bus Selector/1 -> Button Status/1  "<calibration_button_bits>"

== system EMC_no_hand/DataLogging/Keep alive ==
  note: Every 100ms this sends out a message that
      | DexDisplay should get and replay to Dex.
      | That is how Dex can tell if DexDisplay is blocked by a firewall.
  Pack : xpcobsoletelib/Utilities/Pack   datatypes={'double'}  byteAlign=1
  Send : xpcrtudplib/Legacy UDP/Send   ipAddress=192.168.0.1  ipPort=50010  localPort=-1  vblLen=on  sampletime=0.1
  Width : Width
  const : Constant  Value=[1 1 1 1 1]  OutDataTypeStr=double
  wires:
  const/1 -> Pack/1
  Pack/1 -> Width/1, Send/1
  Width/1 -> Send/2

== system EMC_no_hand/DataLogging/Network Transfer Subsystem ==
  note: This subsystem controls the assembly, buffering, and sending of data packets, as well as the receipt of acknowledgements (ACKs). The data packing subsystem packs
      | together multiple data frames, and when its strobe output is set high the send control machine uses this data to create a new packet in its internal ring buffer. Each
      | packet consists of a tracking number, one or more data frames, and a trailing 0. The latter guarantees that the end of the data can be determined by a 0 found in
      | place of a data frame timestamp.
      |
      | The send control machine will send the next packet in its buffer after an ACK for the previous one is received. If it  will resend a packet if it has not received an ACK
      | after a fixed time, and repeat the send for every elapse of that time. Currently up to 5000 packets - a minimum of 5 seconds and a maximum of 30 seconds of data,
      | depending on frame size - are buffered.
  data_frame : Inport
  global clock : Inport  Port=2
  exam_status : Inport  Port=3
  Bus Creator : BusCreator  Inputs=2
  Data Packing Subsystem : Subsystem  TreatAsAtomicUnit=on  SystemSampleTime=0.001
  Data Type Conversion2 : DataTypeConversion
  Mux1 : Mux  Inputs=3
  Queue Size : DataTypeConversion  OutDataTypeStr=int32  SaturateOnIntegerOverflow=on  RndMeth=Zero
  Rate Transition1 : RateTransition  Integrity=off
  Send Control Machine : Stateflow chart  TreatAsAtomicUnit=on
  Task Clock : DiscretePulseGenerator  PulseType=Time based  Period=BKIN_STEP_TIME * 2  PulseWidth=50  SampleTime=0.0005
  Terminator : Terminator
  Total Timeouts : DataTypeConversion  OutDataTypeStr=int32  SaturateOnIntegerOverflow=on  RndMeth=Zero
  UDP Receiver : Subsystem
  UDP Send Subsystem : Subsystem  TreatAsAtomicUnit=on
  force strobe : Subsystem
  max_packet_id : Constant  Value=8000000  OutDataTypeStr=uint32
  runID : Constant  Value=0  OutDataTypeStr=double
  queue : Outport
  wires:
  Rate Transition1/1 -> Send Control Machine/1(data_in)
  force strobe/1(Out1) -> Mux1/1
  Data Packing Subsystem/1(daq_packet_strobe) -> force strobe/1(In1)
  UDP Send Subsystem/1(total_packets_sent) -> Terminator/1  "packet_counter"
  Queue Size/1 -> Bus Creator/1  "queue_size"
  UDP Receiver/1(ACK_ID) -> Send Control Machine/2(ack_packet_index)
  Send Control Machine/2(data_out) -> UDP Send Subsystem/1(packet_data)
  Send Control Machine/5(e_send()) -> UDP Send Subsystem/Trigger
  global clock/1 -> Mux1/2
  Send Control Machine/3(queue_size) -> Queue Size/1
  Send Control Machine/4(total_timeouts) -> Total Timeouts/1
  Mux1/1 -> Send Control Machine/Trigger
  Data Packing Subsystem/2(packed_data) -> Rate Transition1/1
  data_frame/1 -> Data Packing Subsystem/1(data_frame)
  Total Timeouts/1 -> Bus Creator/2  "timeouts"
  max_packet_id/1 -> Send Control Machine/3(max_packet_id)
  runID/1 -> Data Type Conversion2/1
  Data Type Conversion2/1 -> Send Control Machine/4(runID)
  Task Clock/1 -> Mux1/3
  Send Control Machine/1(resetUDP) -> [reset_UDP]
  exam_status/1 -> Send Control Machine/5(is_exam_running)
  [reset_UDP] -> UDP Receiver/1(Trigger UDP reset)
  Bus Creator/1 -> queue/1

== system EMC_no_hand/DataLogging/Poll Force Plates ==
  Convert1 : DataTypeConversion  OutDataTypeStr=uint8
  Convert19 : DataTypeConversion  OutDataTypeStr=double
  Mux2 : Mux  Inputs=6
  Rate Transition : RateTransition  Integrity=off
  Rate Transition1 : RateTransition  Integrity=off
  ain_offset1 : Constant  Value=-1
  ain_offset2 : Constant  Value=-1
  ain_slope1 : Constant  Value=-1
  ain_slope2 : Constant  Value=-1
  calibration_matrix1 : Constant  Value=zeros(6,8)
  calibration_matrix2 : Constant  Value=zeros(6,8)
  enable_plate1 : Constant  Value=0  SampleTime=BKIN_STEP_TIME
  enable_plate2 : Constant  Value=0  SampleTime=BKIN_STEP_TIME
  gain : Constant  Value=256
  orientation1 : Constant  Value=0
  orientation2 : Constant  Value=0
  plate1 : Subsystem
  plate2 : Subsystem
  request_packet : Constant  Value=zeros(1, 34, 'int32')  SampleTime=0.0005
  send poll 1 : Subsystem
  send poll 2 : Subsystem
  zero_voltage : Constant  Value=0
  force plate data : Outport
  wires:
  gain/1 -> plate2/1(gain), plate1/1(gain)
  plate1/1(Forces P1) -> Mux2/1
  plate1/2(Moments P1) -> Mux2/2
  plate1/3(Timer P1) -> Mux2/3
  plate2/1(Forces P1) -> Mux2/4
  plate2/2(Moments P1) -> Mux2/5
  plate2/3(Timer P1) -> Mux2/6
  calibration_matrix1/1 -> plate1/2(calib_matrix)
  calibration_matrix2/1 -> plate2/2(calib_matrix)
  enable_plate1/1 -> plate1/Enable, [plate1]
  enable_plate2/1 -> plate2/Enable, [plate2]
  Mux2/1 -> Convert19/1
  ain_slope1/1 -> plate1/3(ain_slope)
  ain_offset1/1 -> plate1/4(ain_offset)
  ain_slope2/1 -> plate2/3(ain_slope)
  ain_offset2/1 -> plate2/4(ain_offset)
  orientation1/1 -> plate1/5(orientation)
  orientation2/1 -> plate2/5(orientation)
  Convert19/1 -> force plate data/1
  request_packet/1 -> Convert1/1
  zero_voltage/1 -> plate1/6(zero_voltage), plate2/6(zero_voltage)
  Convert1/1 -> send poll 1/1(send packet), send poll 2/1(send packet)
  Rate Transition1/1 -> send poll 2/Enable
  [plate1] -> Rate Transition/1
  [plate2] -> Rate Transition1/1
  Rate Transition/1 -> send poll 1/Enable

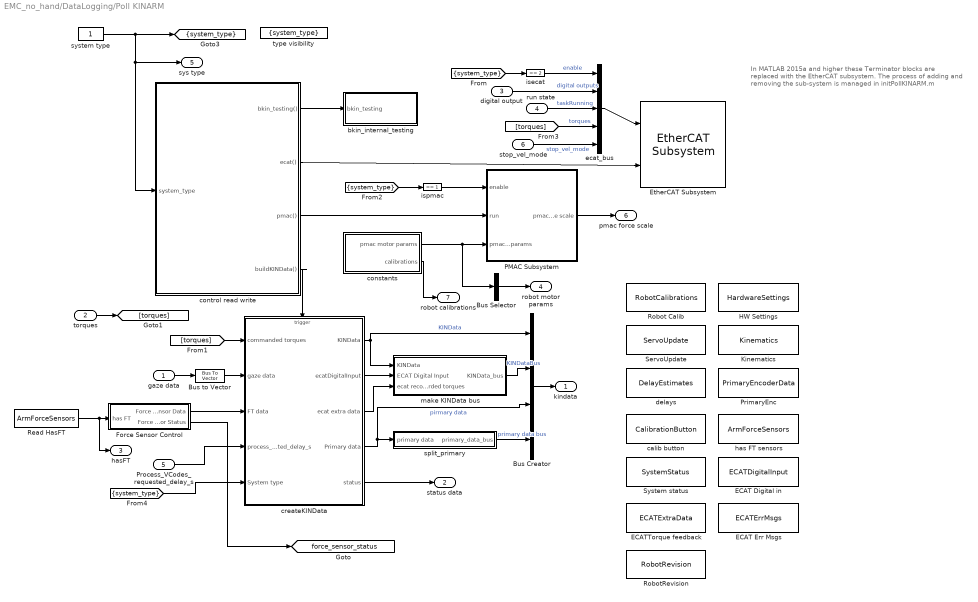
== system EMC_no_hand/DataLogging/Poll KINARM ==
  note: In MATLAB 2015a and higher these Terminator blocks
      | are replaced with the EtherCAT subsystem. The process of
      | adding and removing the sub-system is managed in
      | initPollKINARM.m
  gaze data : Inport
  torques : Inport  Port=2
  digital output : Inport  Port=3
  run state : Inport  Port=4
  Process_VCodes_requested_delay_s : Inport  Port=5
  stop_vel_mode : Inport  Port=6
  Bus Creator : BusCreator
  Bus Selector : BusSelector  OutputSignals=robot1MotorParams,robot2MotorParams  OutputAsBus=on
  Bus to Vector : BusToVector
  ECAT Digital in : DataStoreMemory  DataStoreName=ECATDigitalInput  ReadBeforeWriteMsg=error  WriteAfterWriteMsg=warning  WriteAfterReadMsg=error  InitialValue=[0, 0, 0, 0, 0, 0, 0, 0]  OutDataTypeStr=uint32
  ECAT Err Msgs : DataStoreMemory  DataStoreName=ECATErrMsgs  ReadBeforeWriteMsg=error  WriteAfterWriteMsg=warning  WriteAfterReadMsg=error  InitialValue=zeros(4, 5)  OutDataTypeStr=double
  ECATTorque feedback : DataStoreMemory  DataStoreName=ECATExtraData  ReadBeforeWriteMsg=error  WriteAfterWriteMsg=warning  WriteAfterReadMsg=error  InitialValue=[0, 0, 0, 0, 0, 0, 0, 0, 0, 0]  OutDataTypeStr=double
  EtherCAT Subsystem : ethercat/EtherCAT Subsystem  SystemSampleTime=BKIN_STEP_TIME
  Force Sensor Control : Subsystem  TreatAsAtomicUnit=on
      settings: RTWSystemCode=Nonreusable function  RTWFileNameOpts=Use function name
  HW Settings : DataStoreMemory  DataStoreName=HardwareSettings  ReadBeforeWriteMsg=error  WriteAfterWriteMsg=warning  WriteAfterReadMsg=error  InitialValue=zeros(24, 1)  OutDataTypeStr=double
  Kinematics : DataStoreMemory  DataStoreName=Kinematics  ReadBeforeWriteMsg=error  WriteAfterWriteMsg=warning  WriteAfterReadMsg=error  InitialValue=zeros(20, 1)  OutDataTypeStr=double
  PMAC Subsystem : Subsystem
      settings: RTWSystemCode=Nonreusable function  RTWFileNameOpts=Use function name
  PrimaryEnc : DataStoreMemory  DataStoreName=PrimaryEncoderData  ReadBeforeWriteMsg=error  WriteAfterWriteMsg=warning  WriteAfterReadMsg=error  InitialValue=zeros(12, 1)  OutDataTypeStr=double
  Read HasFT : DataStoreRead  DataStoreName=ArmForceSensors  SampleTime=BKIN_STEP_TIME
  Robot Calib : DataStoreMemory  DataStoreName=RobotCalibrations  InitialValue=zeros(16, 1)  OutDataTypeStr=double
  RobotRevision : DataStoreMemory  DataStoreName=RobotRevision  ReadBeforeWriteMsg=error  WriteAfterWriteMsg=warning  WriteAfterReadMsg=error  InitialValue=[1, 1]  OutDataTypeStr=double
  ServoUpdate : DataStoreMemory  DataStoreName=ServoUpdate  ReadBeforeWriteMsg=error  WriteAfterWriteMsg=warning  WriteAfterReadMsg=error  OutDataTypeStr=uint32
  System status : DataStoreMemory  DataStoreName=SystemStatus  ReadBeforeWriteMsg=error  WriteAfterWriteMsg=warning  WriteAfterReadMsg=error  InitialValue=zeros(1, 7)  OutDataTypeStr=uint32
  bkin_internal_testing : Subsystem
  calib button : DataStoreMemory  DataStoreName=CalibrationButton  ReadBeforeWriteMsg=error  WriteAfterWriteMsg=warning  WriteAfterReadMsg=error  OutDataTypeStr=uint32
  constants : Subsystem
      settings: RTWSystemCode=Nonreusable function  RTWFileNameOpts=Use function name
  control read write : Stateflow chart  TreatAsAtomicUnit=on
  createKINData : Subsystem
      settings: RTWSystemCode=Nonreusable function  RTWFileNameOpts=Use function name
  delays : DataStoreMemory  DataStoreName=DelayEstimates  ReadBeforeWriteMsg=error  WriteAfterWriteMsg=warning  WriteAfterReadMsg=error  InitialValue=zeros(4, 1)  OutDataTypeStr=double
  ecat_bus : BusCreator  Inputs=5
  has FT sensors : DataStoreMemory  DataStoreName=ArmForceSensors  InitialValue=[0, 0]  OutDataTypeStr=double
  isecat : simulink/Logic and Bit Operations/Compare To Constant  relop===  const=2  OutDataTypeStr=boolean
  ispmac : simulink/Logic and Bit Operations/Compare To Constant  relop===  const=1  OutDataTypeStr=boolean
  make KINData bus : Subsystem
  split_primary : Subsystem
  system type : Constant
  type visibility : GotoTagVisibility  GotoTag=system_type
  kindata : Outport
  status data : Outport  Port=2
  hasFT : Outport  Port=3
  robot motor params : Outport  Port=4
  sys type : Outport  Port=5
  pmac force scale : Outport  Port=6
  robot calibrations : Outport  Port=7
  tag scope: force_sensor_status=global, system_type=scoped
  wires:
  control read write/2(ecat()) -> EtherCAT Subsystem/2
  ecat_bus/1 -> EtherCAT Subsystem/1
  stop_vel_mode/1 -> ecat_bus/5  "stop_vel_mode"
  Bus Selector/1 -> robot motor params/1
  Bus Creator/1 -> kindata/1
  Bus to Vector/1 -> createKINData/2(gaze data)
  constants/1(pmac motor params) -> Bus Selector/1, PMAC Subsystem/3(pmac robot params)
  createKINData/1(KINData) -> Bus Creator/1, make KINData bus/1(KINData)  "KINData"
  createKINData/4(Primary data) -> Bus Creator/3, split_primary/1(primary data)  "pirmary data"
  createKINData/5(status) -> status data/1
  gaze data/1 -> Bus to Vector/1
  Force Sensor Control/1(Force Sensor Data) -> createKINData/3(FT data)
  system type/1 -> [system_type], control read write/1(system_type), sys type/1
  control read write/1(bkin_testing()) -> bkin_internal_testing/1(bkin_testing)
  control read write/3(pmac()) -> PMAC Subsystem/2(run)
  control read write/4(buildKINData()) -> createKINData/Trigger
  [system_type] -> isecat/1
  [system_type] -> ispmac/1
  ispmac/1 -> PMAC Subsystem/1(enable)
  Read HasFT/1 -> hasFT/1, Force Sensor Control/1(has FT)
  make KINData bus/1(KINData_bus) -> Bus Creator/2  "KINDataBus"
  split_primary/1(primary_data_bus) -> Bus Creator/4  "primary data bus"
  PMAC Subsystem/1(pmac force scale) -> pmac force scale/1
  constants/2(calibrations) -> robot calibrations/1
  createKINData/2(ecatDigitalInput) -> make KINData bus/2(ECAT Digital Input)
  digital output/1 -> ecat_bus/2  "digital outputs"
  run state/1 -> ecat_bus/3  "taskRunning"
  isecat/1 -> ecat_bus/1  "enable"
  torques/1 -> [torques]
  [torques] -> createKINData/1(commanded torques)
  [torques] -> ecat_bus/4  "torques"
  createKINData/3(ecat extra data) -> make KINData bus/3(ecat recorded torques)
  Process_VCodes_requested_delay_s/1 -> createKINData/4(process_vcodes_requested_delay_s)
  Force Sensor Control/2(Force Sensor Status) -> [force_sensor_status]
  [system_type] -> createKINData/5(System type)
